simulink model "Problem_16_4"  (Simulink 7.5)
settings: Solver=ode45  StartTime=0.0  StopTime=10.0  RelTol=1e-3
settings Model: Creator=Holly  LastModifiedBy=Holly

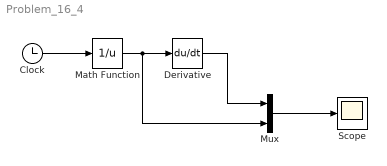
== system Problem_16_4 ==
  Clock : Clock
      settings: Decimation=10
  Derivative : Derivative
  Math Function : Math  Operator=reciprocal  OutDataType=fixdt(1, 16)  OutScaling=2^0  SaturateOnIntegerOverflow=on
  Mux : Mux  Inputs=2
  Scope : Scope
  wires:
  Clock/1 -> Math Function/1
  Math Function/1 -> Derivative/1, Mux/2
  Derivative/1 -> Mux/1
  Mux/1 -> Scope/1
